simulink model "solar_wind_system_with_statcom"  (R2024a)
settings: Solver=VariableStepAuto  StartTime=0.0  StopTime=1  RelTol=1e-3
undefined symbols (not defined in the file): DiscIntNeverNeededParam, R
libraries: neural x24, spsSeriesRLCBranchLib x24, spsVoltageMeasurementLib x12, spsDiodeLib x10, powerlib_extras x9, simulink x7, spsIGBTDiodeLib x6, spsCurrentMeasurementLib x5, spsThreePhaseVIMeasurementLib x4, spsBreakerLib x3, spsPower3phInstantaneousLib x3, spsControlledCurrentSourceLib x3
(part 3 of 3)

== system solar_wind_system_with_statcom/Feed-Forward Neural Network2/Layer 2/LW{2,1} ==
  "ad{2,1}" : Inport  PortDimensions=3
      mask Display: e = 0.06;c1 = [120 230 180]/255;c2 = ([120 230 180]+0)/(256+128);c3 = ([120 230 180]+128)/(256+128);patch([0 1 1 0],[0 0 1 1],c1);patch([0 1 1 1-e 1-e 0+e],[0 0 1 1-e 0+e 0+e],c2);patch([0 0 1 1-e 0+e 0+e],[0 1 1 1-e 1-e 0+e],c3);plot([0 1 1 0 0],[0 0 1 1 0]);
  "IW{2,1}(1,:)'" : Constant  Value=[-11.0653035405260151691209102864377200603485107421875;-0.1255372019525728133348962956006289459764957427978515625;-0.372892044827420832131537054010550491511821746826171875]
      mask Display: e = 0.06;c1 = [120 150 230]/255;c2 = ([120 150 230]+0)/383;c3 = ([120 150 230]+128)/383;patch([0 1 1 0],[0 0 1 1],c1);patch([0 1 1 1-e 1-e 0+e],[0 0 1 1-e 0+e 0+e],c2);patch([0 0 1 1-e 0+e 0+e],[0 1 1 1-e 1-e 0+e],c3);plot([0 1 1 0 0],[0 0 1 1 0]);disp('weights');
  Mux : Mux  Inputs=1
      mask Display: e = 0.06;c1 = [120 150 230]/255;c2 = ([120 150 230]+0)/383;c3 = ([120 150 230]+128)/383;patch([0 1 1 0],[0 0 1 1],c1);patch([0 1 1 1-e 1-e 0+e],[0 0 1 1-e 0+e 0+e],c2);patch([0 0 1 1-e 0+e 0+e],[0 1 1 1-e 1-e 0+e],c3);plot([0 1 1 0 0],[0 0 1 1 0]);disp('Mux');
  dotprod1 : neural/Weight Functions/dotprod
  "lz{2,1}" : Outport
      mask Display: e = 0.06;c1 = [120 230 180]/255;c2 = ([120 230 180]+0)/(256+128);c3 = ([120 230 180]+128)/(256+128);patch([0 1 1 0],[0 0 1 1],c1);patch([0 1 1 1-e 1-e 0+e],[0 0 1 1-e 0+e 0+e],c2);patch([0 0 1 1-e 0+e 0+e],[0 1 1 1-e 1-e 0+e],c3);plot([0 1 1 0 0],[0 0 1 1 0]);
  wires:
  "IW{2,1}(1,:)'"/1 -> dotprod1/1
  "ad{2,1}"/1 -> dotprod1/2
  dotprod1/1 -> Mux/1
  Mux/1 -> "lz{2,1}"/1

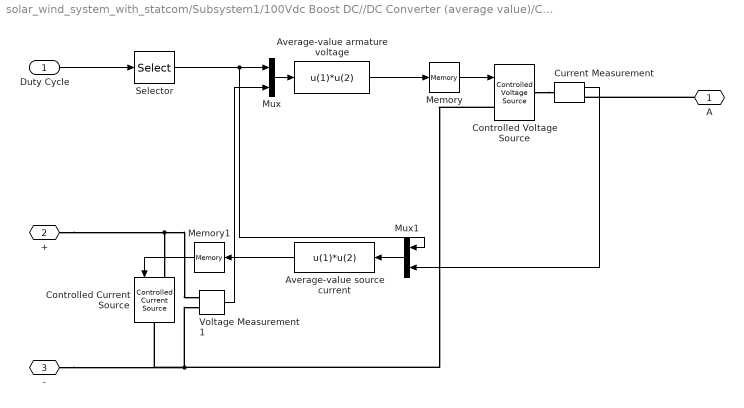
== system solar_wind_system_with_statcom/Subsystem1/100Vdc Boost DC//DC Converter (average value)/Chopper ==
  Duty Cycle : Inport
  Average-value armature voltage : Fcn  Expr=u(1)*u(2)
  Average-value source current : Fcn  Expr=u(1)*u(2)
  Controlled Current Source : spsControlledCurrentSourceLib/Controlled Current Source  Initialize=on  Source_Type=AC  Amplitude=0  Phase=0  Frequency=0  Measurements=None
  Controlled Voltage Source : spsControlledVoltageSourceLib/Controlled Voltage Source  Initialize=on  Source_Type=AC  Amplitude=0  Phase=0  Frequency=0  Measurements=None
  Current Measurement : spsCurrentMeasurementLib/Current Measurement  Tag=PoWeRsYsTeMmEaSuReMeNt  PhasorSimulation=off  OutputType=Magnitude  PSBequivalent=0
      settings: AttributesFormatString=\n
  Memory : Memory
  Memory1 : Memory
  Mux : Mux  Inputs=2
  Mux1 : Mux  Inputs=2
  Selector : Selector  InputPortWidth=2  IndexOptions=Index vector (dialog)  Indices=[1]  OutputSizes=1
  Voltage Measurement1 : spsVoltageMeasurementLib/Voltage Measurement  Tag=PoWeRsYsTeMmEaSuReMeNt  PhasorSimulation=off  OutputType=Magnitude  PSBequivalent=0
  A : PMIOPort  Side=Right
  + : PMIOPort  Port=2  Side=Left
  - : PMIOPort  Port=3  Side=Left
  wires:
  Selector/1 -> Mux1/1, Mux/1
  Memory1/1 -> Controlled Current Source/1
  Average-value source current/1 -> Memory1/1
  Current Measurement/1 -> Mux1/2
  Mux1/1 -> Average-value source current/1
  Duty Cycle/1 -> Selector/1
  Voltage Measurement1/1 -> Mux/2
  Mux/1 -> Average-value armature voltage/1
  Average-value armature voltage/1 -> Memory/1
  Memory/1 -> Controlled Voltage Source/1
  connections:
  A/RConn1 -- Current Measurement/RConn1
  Controlled Voltage Source/RConn1 -- Current Measurement/LConn1
  +/RConn1 -- Voltage Measurement1/LConn1 -- Controlled Current Source/LConn1
  Controlled Voltage Source/LConn1 -- -/RConn1 -- Controlled Current Source/RConn1 -- Voltage Measurement1/LConn2

== system solar_wind_system_with_statcom/Subsystem1/100Vdc Boost DC//DC Converter (average value)/Current controller DISCRETE1 ==
  UBus : Inport
  Uref : Inport  Port=2
  Ctrl sat. : Saturate  UpperLimit=0.95  LowerLimit=-0.95
  Discrete-Time Integrator : DiscreteIntegrator  IntegratorMethod=Integration: Trapezoidal  SampleTime=Ts  LimitOutput=on  UpperSaturationLimit=0.95  LowerSaturationLimit=-0.95  ICPrevOutput=DiscIntNeverNeededParam  ICPrevScaledInput=DiscIntNeverNeededParam
  Integral gain : Gain  Gain=Ki  SaturateOnIntegerOverflow=on  OutDataTypeStr=Inherit: Same as input  ParamDataTypeStr=Inherit: Same as input
  Proportional gain : Gain  Gain=Kp  SaturateOnIntegerOverflow=on  OutDataTypeStr=Inherit: Same as input  ParamDataTypeStr=Inherit: Same as input
  Sum1 : Sum  Inputs=+-  InputSameDT=on  SaturateOnIntegerOverflow=on  OutDataTypeStr=Inherit: Same as first input
  Sum2 : Sum  InputSameDT=on  SaturateOnIntegerOverflow=on  OutDataTypeStr=Inherit: Same as first input
  Ec : Outport  InitialOutput=0
  wires:
  Ctrl sat./1 -> Ec/1
  Sum2/1 -> Ctrl sat./1
  Discrete-Time Integrator/1 -> Sum2/2
  Uref/1 -> Sum1/2
  UBus/1 -> Sum1/1
  Sum1/1 -> Proportional gain/1, Integral gain/1
  Integral gain/1 -> Discrete-Time Integrator/1
  Proportional gain/1 -> Sum2/1

== system solar_wind_system_with_statcom/Subsystem1/100Vdc Boost DC//DC Converter (average value)/Duty Cycles ==
  Ec : Inport
  Add : Sum  Inputs=+-
  Bus Creator2 : BusCreator  Inputs=2
  Constant : Constant
  Duty Cycle : Fcn  Expr=0.5*(u[1]+1)
  dc : Outport
  wires:
  Bus Creator2/1 -> dc/1
  Ec/1 -> Duty Cycle/1
  Constant/1 -> Add/1
  Add/1 -> Bus Creator2/2  "IGBT 2"
  Duty Cycle/1 -> Bus Creator2/1, Add/2  "IGBT I"

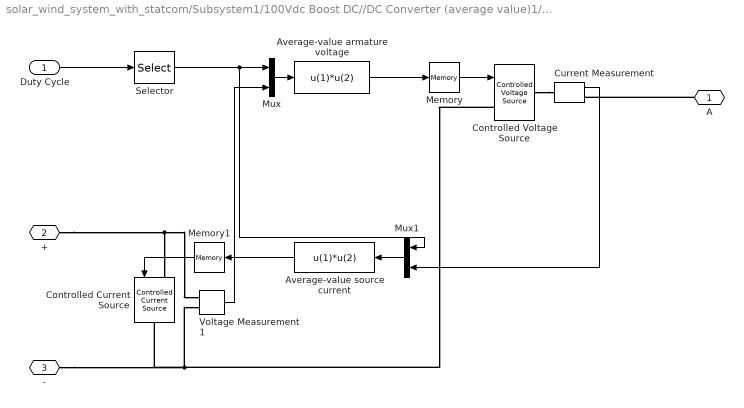
== system solar_wind_system_with_statcom/Subsystem1/100Vdc Boost DC//DC Converter (average value)1/Chopper ==
  Duty Cycle : Inport
  Average-value armature voltage : Fcn  Expr=u(1)*u(2)
  Average-value source current : Fcn  Expr=u(1)*u(2)
  Controlled Current Source : spsControlledCurrentSourceLib/Controlled Current Source  Initialize=on  Source_Type=AC  Amplitude=0  Phase=0  Frequency=0  Measurements=None
  Controlled Voltage Source : spsControlledVoltageSourceLib/Controlled Voltage Source  Initialize=on  Source_Type=AC  Amplitude=0  Phase=0  Frequency=0  Measurements=None
  Current Measurement : spsCurrentMeasurementLib/Current Measurement  Tag=PoWeRsYsTeMmEaSuReMeNt  PhasorSimulation=off  OutputType=Magnitude  PSBequivalent=0
      settings: AttributesFormatString=\n
  Memory : Memory
  Memory1 : Memory
  Mux : Mux  Inputs=2
  Mux1 : Mux  Inputs=2
  Selector : Selector  InputPortWidth=2  IndexOptions=Index vector (dialog)  Indices=[1]  OutputSizes=1
  Voltage Measurement1 : spsVoltageMeasurementLib/Voltage Measurement  Tag=PoWeRsYsTeMmEaSuReMeNt  PhasorSimulation=off  OutputType=Magnitude  PSBequivalent=0
  A : PMIOPort  Side=Right
  + : PMIOPort  Port=2  Side=Left
  - : PMIOPort  Port=3  Side=Left
  wires:
  Selector/1 -> Mux1/1, Mux/1
  Memory1/1 -> Controlled Current Source/1
  Average-value source current/1 -> Memory1/1
  Current Measurement/1 -> Mux1/2
  Mux1/1 -> Average-value source current/1
  Duty Cycle/1 -> Selector/1
  Voltage Measurement1/1 -> Mux/2
  Mux/1 -> Average-value armature voltage/1
  Average-value armature voltage/1 -> Memory/1
  Memory/1 -> Controlled Voltage Source/1
  connections:
  A/RConn1 -- Current Measurement/RConn1
  Controlled Voltage Source/RConn1 -- Current Measurement/LConn1
  +/RConn1 -- Voltage Measurement1/LConn1 -- Controlled Current Source/LConn1
  Controlled Voltage Source/LConn1 -- -/RConn1 -- Controlled Current Source/RConn1 -- Voltage Measurement1/LConn2

== system solar_wind_system_with_statcom/Subsystem1/100Vdc Boost DC//DC Converter (average value)1/Current controller DISCRETE1 ==
  UBus : Inport
  Uref : Inport  Port=2
  Ctrl sat. : Saturate  UpperLimit=0.95  LowerLimit=-0.95
  Discrete-Time Integrator : DiscreteIntegrator  IntegratorMethod=Integration: Trapezoidal  SampleTime=Ts  LimitOutput=on  UpperSaturationLimit=0.95  LowerSaturationLimit=-0.95  ICPrevOutput=DiscIntNeverNeededParam  ICPrevScaledInput=DiscIntNeverNeededParam
  Integral gain : Gain  Gain=Ki  SaturateOnIntegerOverflow=on  OutDataTypeStr=Inherit: Same as input  ParamDataTypeStr=Inherit: Same as input
  Proportional gain : Gain  Gain=Kp  SaturateOnIntegerOverflow=on  OutDataTypeStr=Inherit: Same as input  ParamDataTypeStr=Inherit: Same as input
  Sum1 : Sum  Inputs=+-  InputSameDT=on  SaturateOnIntegerOverflow=on  OutDataTypeStr=Inherit: Same as first input
  Sum2 : Sum  InputSameDT=on  SaturateOnIntegerOverflow=on  OutDataTypeStr=Inherit: Same as first input
  Ec : Outport  InitialOutput=0
  wires:
  Ctrl sat./1 -> Ec/1
  Sum2/1 -> Ctrl sat./1
  Discrete-Time Integrator/1 -> Sum2/2
  Uref/1 -> Sum1/2
  UBus/1 -> Sum1/1
  Sum1/1 -> Proportional gain/1, Integral gain/1
  Integral gain/1 -> Discrete-Time Integrator/1
  Proportional gain/1 -> Sum2/1

== system solar_wind_system_with_statcom/Subsystem1/100Vdc Boost DC//DC Converter (average value)1/Duty Cycles ==
  Ec : Inport
  Add : Sum  Inputs=+-
  Bus Creator2 : BusCreator  Inputs=2
  Constant : Constant
  Duty Cycle : Fcn  Expr=0.5*(u[1]+1)
  dc : Outport
  wires:
  Bus Creator2/1 -> dc/1
  Ec/1 -> Duty Cycle/1
  Constant/1 -> Add/1
  Add/1 -> Bus Creator2/2  "IGBT 2"
  Duty Cycle/1 -> Bus Creator2/1, Add/2  "IGBT I"

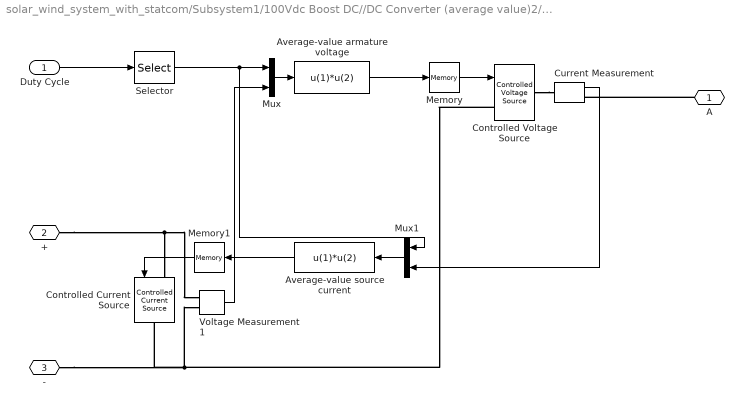
== system solar_wind_system_with_statcom/Subsystem1/100Vdc Boost DC//DC Converter (average value)2/Chopper ==
  Duty Cycle : Inport
  Average-value armature voltage : Fcn  Expr=u(1)*u(2)
  Average-value source current : Fcn  Expr=u(1)*u(2)
  Controlled Current Source : spsControlledCurrentSourceLib/Controlled Current Source  Initialize=on  Source_Type=AC  Amplitude=0  Phase=0  Frequency=0  Measurements=None
  Controlled Voltage Source : spsControlledVoltageSourceLib/Controlled Voltage Source  Initialize=on  Source_Type=AC  Amplitude=0  Phase=0  Frequency=0  Measurements=None
  Current Measurement : spsCurrentMeasurementLib/Current Measurement  Tag=PoWeRsYsTeMmEaSuReMeNt  PhasorSimulation=off  OutputType=Magnitude  PSBequivalent=0
      settings: AttributesFormatString=\n
  Memory : Memory
  Memory1 : Memory
  Mux : Mux  Inputs=2
  Mux1 : Mux  Inputs=2
  Selector : Selector  InputPortWidth=2  IndexOptions=Index vector (dialog)  Indices=[1]  OutputSizes=1
  Voltage Measurement1 : spsVoltageMeasurementLib/Voltage Measurement  Tag=PoWeRsYsTeMmEaSuReMeNt  PhasorSimulation=off  OutputType=Magnitude  PSBequivalent=0
  A : PMIOPort  Side=Right
  + : PMIOPort  Port=2  Side=Left
  - : PMIOPort  Port=3  Side=Left
  wires:
  Selector/1 -> Mux1/1, Mux/1
  Memory1/1 -> Controlled Current Source/1
  Average-value source current/1 -> Memory1/1
  Current Measurement/1 -> Mux1/2
  Mux1/1 -> Average-value source current/1
  Duty Cycle/1 -> Selector/1
  Voltage Measurement1/1 -> Mux/2
  Mux/1 -> Average-value armature voltage/1
  Average-value armature voltage/1 -> Memory/1
  Memory/1 -> Controlled Voltage Source/1
  connections:
  A/RConn1 -- Current Measurement/RConn1
  Controlled Voltage Source/RConn1 -- Current Measurement/LConn1
  +/RConn1 -- Voltage Measurement1/LConn1 -- Controlled Current Source/LConn1
  Controlled Voltage Source/LConn1 -- -/RConn1 -- Controlled Current Source/RConn1 -- Voltage Measurement1/LConn2

== system solar_wind_system_with_statcom/Subsystem1/100Vdc Boost DC//DC Converter (average value)2/Current controller DISCRETE1 ==
  UBus : Inport
  Uref : Inport  Port=2
  Ctrl sat. : Saturate  UpperLimit=0.95  LowerLimit=-0.95
  Discrete-Time Integrator : DiscreteIntegrator  IntegratorMethod=Integration: Trapezoidal  SampleTime=Ts  LimitOutput=on  UpperSaturationLimit=0.95  LowerSaturationLimit=-0.95  ICPrevOutput=DiscIntNeverNeededParam  ICPrevScaledInput=DiscIntNeverNeededParam
  Integral gain : Gain  Gain=Ki  SaturateOnIntegerOverflow=on  OutDataTypeStr=Inherit: Same as input  ParamDataTypeStr=Inherit: Same as input
  Proportional gain : Gain  Gain=Kp  SaturateOnIntegerOverflow=on  OutDataTypeStr=Inherit: Same as input  ParamDataTypeStr=Inherit: Same as input
  Sum1 : Sum  Inputs=+-  InputSameDT=on  SaturateOnIntegerOverflow=on  OutDataTypeStr=Inherit: Same as first input
  Sum2 : Sum  InputSameDT=on  SaturateOnIntegerOverflow=on  OutDataTypeStr=Inherit: Same as first input
  Ec : Outport  InitialOutput=0
  wires:
  Ctrl sat./1 -> Ec/1
  Sum2/1 -> Ctrl sat./1
  Discrete-Time Integrator/1 -> Sum2/2
  Uref/1 -> Sum1/2
  UBus/1 -> Sum1/1
  Sum1/1 -> Proportional gain/1, Integral gain/1
  Integral gain/1 -> Discrete-Time Integrator/1
  Proportional gain/1 -> Sum2/1

== system solar_wind_system_with_statcom/Subsystem1/100Vdc Boost DC//DC Converter (average value)2/Duty Cycles ==
  Ec : Inport
  Add : Sum  Inputs=+-
  Bus Creator2 : BusCreator  Inputs=2
  Constant : Constant
  Duty Cycle : Fcn  Expr=0.5*(u[1]+1)
  dc : Outport
  wires:
  Bus Creator2/1 -> dc/1
  Ec/1 -> Duty Cycle/1
  Constant/1 -> Add/1
  Add/1 -> Bus Creator2/2  "IGBT 2"
  Duty Cycle/1 -> Bus Creator2/1, Add/2  "IGBT I"

== matlab function solar_wind_system_with_statcom/Subsystem1/MATLAB Function ==
  data: fuelcell_current input; output output
function output = fuzzy_sugeno_affc3(fuelcell_current)
    % Define the membership function parameters for Fuelcell__Current
    in1mf1_params = [-30 30 90];    % trimf for in1mf1
    in1mf2_params = [30 90 150];    % trimf for in1mf2
    in1mf3_params = [90 150 210];   % trimf for in1mf3
    
    % Evaluate membership functions for Fuelcell__Current
    in1mf1 = trimf(fuelcell_current, in1mf1_params);  % Membership value for in1mf1
    in1mf2 = trimf(fuelcell_current, in1mf2_params);  % Membership value for in1mf2
    in1mf3 = trimf(fuelcell_current, in1mf3_params);  % Membership value for in1mf3
    
    % Define rule outputs (constant values for Flow__Control)
    output1 = 48.8999987975491;  % out1mf1
    output2 = 48.2999999900248;  % out1mf2
    output3 = 47.6999988271882;  % out1mf3
    
    % Initialize output to NaN (in case no rule is fired)
    output = NaN;
    
    % Rule 1: If Fuelcell__Current is in1mf1, then Flow__Control is out1mf1
    if in1mf1 > 0
        output = output1;
    end
    
    % Rule 2: If Fuelcell__Current is in1mf2, then Flow__Control is out1mf2
    if in1mf2 > 0
        output = output2;
    end
    
    % Rule 3: If Fuelcell__Current is in1mf3, then Flow__Control is out1mf3
    if in1mf3 > 0
        output = output3;
    end
    
    % Handling of overlapping conditions (if multiple rules fire)
    % Using weighted average method (wtaver as defuzzification method)
    if (in1mf1 > 0) && (in1mf2 > 0) || (in1mf2 > 0) && (in1mf3 > 0)
        output = (in1mf1 * output1 + in1mf2 * output2 + in1mf3 * output3) / ...
                 (in1mf1 + in1mf2 + in1mf3);
    end
end

== matlab function solar_wind_system_with_statcom/Wind 3kW Poweer System/MATLAB Function ==
  data: V_w input; dutyCycle output; I_w input
function dutyCycle = POMPPT(V_w, I_w)
    % P&O MPPT algorithm for PV systems

    persistent previousPower
    persistent perturbDirection

    % Parameters
    stepSize = 0.01;  % Perturbation step size

    % Calculate instantaneous power
    power = V_w * I_w;

    % Initialize variables on the first run
    if isempty(previousPower)
        previousPower = power;
        perturbDirection = 1;  % 1 for perturb up, -1 for perturb down
    end

    % Compare current power with previous power
    if power > previousPower
        % If power increased, continue perturbing in the same direction
        dutyCycle = perturbDirection * stepSize + previousPower;
    else
        % If power decreased, change perturbation direction
        perturbDirection = -perturbDirection;
        dutyCycle = previousPower;
    end

    % Update previous power for the next iteration
    previousPower = power;

    % Ensure duty cycle is within [0, 1] range
    dutyCycle = max(0, min(1, dutyCycle));
end

== matlab function solar_wind_system_with_statcom/Subsystem1/MATLAB Function1 ==
  data: fuelcell_current input; output output
function output = fuzzy_sugeno_affc3(fuelcell_current)
    % Define the membership function parameters for Fuelcell__Current
    in1mf1_params = [-30 30 90];    % trimf for in1mf1
    in1mf2_params = [30 90 150];    % trimf for in1mf2
    in1mf3_params = [90 150 210];   % trimf for in1mf3
    
    % Evaluate membership functions for Fuelcell__Current
    in1mf1 = trimf(fuelcell_current, in1mf1_params);  % Membership value for in1mf1
    in1mf2 = trimf(fuelcell_current, in1mf2_params);  % Membership value for in1mf2
    in1mf3 = trimf(fuelcell_current, in1mf3_params);  % Membership value for in1mf3
    
    % Define rule outputs (constant values for Flow__Control)
    output1 = 48.8999987975491;  % out1mf1
    output2 = 48.2999999900248;  % out1mf2
    output3 = 47.6999988271882;  % out1mf3
    
    % Initialize output to NaN (in case no rule is fired)
    output = NaN;
    
    % Rule 1: If Fuelcell__Current is in1mf1, then Flow__Control is out1mf1
    if in1mf1 > 0
        output = output1;
    end
    
    % Rule 2: If Fuelcell__Current is in1mf2, then Flow__Control is out1mf2
    if in1mf2 > 0
        output = output2;
    end
    
    % Rule 3: If Fuelcell__Current is in1mf3, then Flow__Control is out1mf3
    if in1mf3 > 0
        output = output3;
    end
    
    % Handling of overlapping conditions (if multiple rules fire)
    % Using weighted average method (wtaver as defuzzification method)
    if (in1mf1 > 0) && (in1mf2 > 0) || (in1mf2 > 0) && (in1mf3 > 0)
        output = (in1mf1 * output1 + in1mf2 * output2 + in1mf3 * output3) / ...
                 (in1mf1 + in1mf2 + in1mf3);
    end
end

== matlab function solar_wind_system_with_statcom/Subsystem1/MATLAB Function2 ==
  data: fuelcell_current input; output output
function output = fuzzy_sugeno_affc3(fuelcell_current)
    % Define the membership function parameters for Fuelcell__Current
    in1mf1_params = [-30 30 90];    % trimf for in1mf1
    in1mf2_params = [30 90 150];    % trimf for in1mf2
    in1mf3_params = [90 150 210];   % trimf for in1mf3
    
    % Evaluate membership functions for Fuelcell__Current
    in1mf1 = trimf(fuelcell_current, in1mf1_params);  % Membership value for in1mf1
    in1mf2 = trimf(fuelcell_current, in1mf2_params);  % Membership value for in1mf2
    in1mf3 = trimf(fuelcell_current, in1mf3_params);  % Membership value for in1mf3
    
    % Define rule outputs (constant values for Flow__Control)
    output1 = 48.8999987975491;  % out1mf1
    output2 = 48.2999999900248;  % out1mf2
    output3 = 47.6999988271882;  % out1mf3
    
    % Initialize output to NaN (in case no rule is fired)
    output = NaN;
    
    % Rule 1: If Fuelcell__Current is in1mf1, then Flow__Control is out1mf1
    if in1mf1 > 0
        output = output1;
    end
    
    % Rule 2: If Fuelcell__Current is in1mf2, then Flow__Control is out1mf2
    if in1mf2 > 0
        output = output2;
    end
    
    % Rule 3: If Fuelcell__Current is in1mf3, then Flow__Control is out1mf3
    if in1mf3 > 0
        output = output3;
    end
    
    % Handling of overlapping conditions (if multiple rules fire)
    % Using weighted average method (wtaver as defuzzification method)
    if (in1mf1 > 0) && (in1mf2 > 0) || (in1mf2 > 0) && (in1mf3 > 0)
        output = (in1mf1 * output1 + in1mf2 * output2 + in1mf3 * output3) / ...
                 (in1mf1 + in1mf2 + in1mf3);
    end
end

== matlab function solar_wind_system_with_statcom/Subsystem2/MATLAB Function ==
  data: V_pv input; dutyCycle output; I_pv input
function dutyCycle = POMPPT(V_pv, I_pv)
    % P&O MPPT algorithm for PV systems

    persistent previousPower
    persistent perturbDirection

    % Parameters
    stepSize = 0.01;  % Perturbation step size

    % Calculate instantaneous power
    power = V_pv * I_pv;

    % Initialize variables on the first run
    if isempty(previousPower)
        previousPower = power;
        perturbDirection = 1;  % 1 for perturb up, -1 for perturb down
    end

    % Compare current power with previous power
    if power > previousPower
        % If power increased, continue perturbing in the same direction
        dutyCycle = perturbDirection * stepSize + previousPower;
    else
        % If power decreased, change perturbation direction
        perturbDirection = -perturbDirection;
        dutyCycle = previousPower;
    end

    % Update previous power for the next iteration
    previousPower = power;

    % Ensure duty cycle is within [0, 1] range
    dutyCycle = max(0, min(1, dutyCycle));
end
